simulink model "car_pendulum_simulation"  (R2017b)
settings: Solver=VariableStepAuto  StartTime=0.0  StopTime=inf  RelTol=1e-3
values from neighbouring files (symbols this model uses):
  A = [0 0 0 1 0 0 ... (first row only)    [DIPV_LQR_gain_calculation.m]    (also in LQR_gain_calculation.m = [0 0       1 0)
  B = [0 ... (first row only)    [DIPV_LQR_gain_calculation.m]    (also in LQR_gain_calculation.m = [0;0;inv(E)*H])
  C = eye(6)    [DIPV_LQR_gain_calculation.m]    (also in LQR_gain_calculation.m = eye(4))
  D = zeros(6,1)    [DIPV_LQR_gain_calculation.m]    (also in LQR_gain_calculation.m = zeros(4,1))
  k0 = k(1)    [DIPV_LQR_gain_calculation.m]    (also in LQR_gain_calculation.m)
  k1 = k(2)    [DIPV_LQR_gain_calculation.m]    (also in LQR_gain_calculation.m)
  k2 = k(3)    [DIPV_LQR_gain_calculation.m]    (also in LQR_gain_calculation.m)
  k3 = k(4)    [DIPV_LQR_gain_calculation.m]    (also in LQR_gain_calculation.m)
libraries: simulink x2
settings Model: Creator=lenovo  LastModifiedBy=lenovo

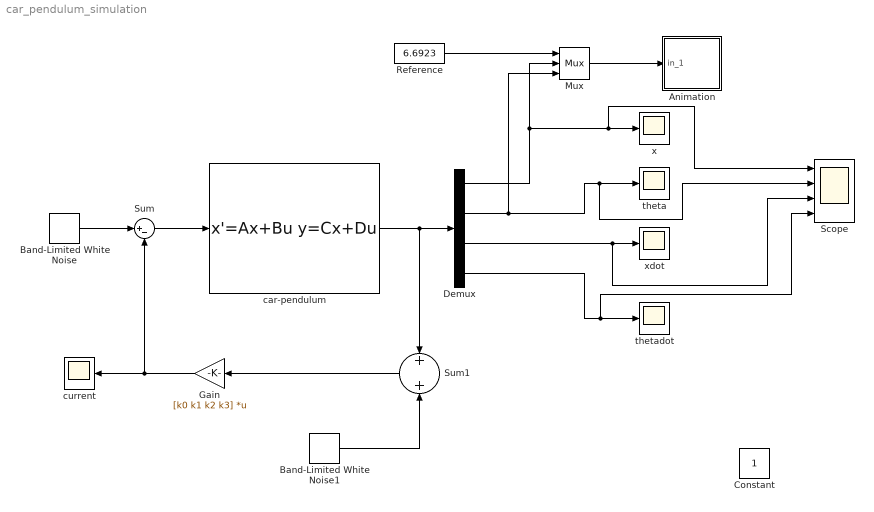
== system car_pendulum_simulation ==
  Animation : Subsystem  mask(Pendulum plot){RefBlock=Reference}
      mask prompts: RefBlock "DC reference signal block name:"
      mask help: Pendulum plot
      mask Help: Pendulum animation function using Handle graphics.
      mask Display: plot([-10 10],[0 0],[-2 -2 2 2],[0 1 1 0],[0 3],[1 5])
  Band-Limited White Noise : simulink/Sources/Band-Limited White Noise  Cov=[0.0000]  Ts=0.01  seed=[23341]
  Band-Limited White Noise1 : simulink/Sources/Band-Limited White Noise  Cov=[0.0000000]  Ts=0.01  seed=[23341]
  Constant : Constant
  Demux : Demux
  Gain : Gain  Gain=[k0 k1 k2 k3]  Multiplication=Matrix(K*u)
  Mux : Mux  Inputs=3
  Reference : Constant  Value=6.6923
  Scope : Scope  NumInputPorts=4
  Sum : Sum  Inputs=|+-
  Sum1 : Sum
  car-pendulum : StateSpace  A=A  B=B  C=C  D=D  InitialCondition=[0 1 0 0]
  current : Scope
  theta : Scope
  thetadot : Scope
  x : Scope
  xdot : Scope
  wires:
  Demux/1 -> Mux/2, Scope/1, x/1
  Demux/2 -> Mux/3, Scope/2, theta/1
  Demux/3 -> Scope/3, xdot/1
  Demux/4 -> Scope/4, thetadot/1
  Mux/1 -> Animation/1(in_1)
  Reference/1 -> Mux/1
  Gain/1 -> current/1, Sum/2
  car-pendulum/1 -> Sum1/1, Demux/1
  Sum/1 -> car-pendulum/1
  Band-Limited White Noise/1 -> Sum/1
  Band-Limited White Noise1/1 -> Sum1/2
  Sum1/1 -> Gain/1

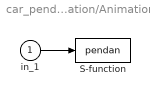
== system car_pendulum_simulation/Animation ==
  in_1 : Inport
  S-function : S-Function  FunctionName=pendan  Parameters=RefBlock  SFunctionDeploymentMode=off  EnableBusSupport=off
      settings: DeleteFcn=pendan([],[],[],'DeleteBlock');
  wires:
  in_1/1 -> S-function/1
